simulink subsystem "i2c_slave_serializer"  (R2022b)
settings: Solver=VariableStepAuto  StartTime=0.0  StopTime=10.0  RelTol=1e-3
libraries: hdlsllib x20, simulink x18
Description:
  | //////////////////////////////////////////////////////////////////////
  | ////                                                              ////
  | //// serialInterface.v                                                 ////
  | ////                                                              ////
  | //// This file is part of the i2cSlave opencores effort.
  | //// <http://www.opencores.org/cores//>                           ////
  | ////                                                              ////
  | //// Module Description:                                          ////
  | //// Perform all serial to parallel, and parallel
  | //// to serial conversions. Perform device address matching
  | //// Handle arbitrary length I2C reads terminated by NAK
  | //// from host, and arbitrary length I2C writes terminated
  | //// by STOP from host
  | //// The second byte of a I2C write is always interpreted
  | //// as a register address, and becomes the base register address
  | //// for all read and write transactions.
  | //// I2C WRITE:    devAddr, regAddr, data[regAddr], data[regAddr+1], ..... data[regAddr+N]
  | //// I2C READ:    data[regAddr], data[regAddr+1], ..... data[regAddr+N]
  | //// Note that when regAddR reaches 255 it will automatically wrap round to 0
  | ////                                                              ////
  | //// To Do:                                                       ////
  | ////
  | ////                                                              ////
  | //// Author(s):                                                   ////
  | //// - Steve Fielding, sfielding@base2designs.com                 ////
  | ////                                                              ////
  | //////////////////////////////////////////////////////////////////////
  | ////                                                              ////
  | //// Copyright (C) 2008 Steve Fielding and OPENCORES.ORG          ////
  | ////                                                              ////
  | //// This source file may be used and distributed without         ////
  | //// restriction provided that this copyright statement is not    ////
  | //// removed from the file and that any derivative work contains  ////
  | //// the original copyright notice and the associated disclaimer. ////
  | ////                                                              ////
  | //// This source file is free software; you can redistribute it   ////
  | //// and/or modify it under the terms of the GNU Lesser General   ////
  | //// Public License as published by the Free Software Foundation; ////
  | //// either version 2.1 of the License, or (at your option) any   ////
  | //// later version.                                               ////
  | ////                                                              ////
  | //// This source is distributed in the hope that it will be       ////
  | //// useful, but WITHOUT ANY WARRANTY; without even the implied   ////
  | //// warranty of MERCHANTABILITY or FITNESS FOR A PARTICULAR      ////
  | //// PURPOSE. See the GNU Lesser General Public License for more  ////
  | //// details.                                                     ////
  | ////                                                              ////
  | //// You should have received a copy of the GNU Lesser General    ////
  | //// Public License along with this source; if not, download it   ////
  | //// from <http://www.opencores.org/lgpl.shtml>                   ////
  | ////                                                              ////
  | //////////////////////////////////////////////////////////////////////
settings Model: Creator=evsenin  LastModifiedBy=evsenin
settings ModelReferenceCC: EnableRefExpFcnMdlSchedulingChecks=on

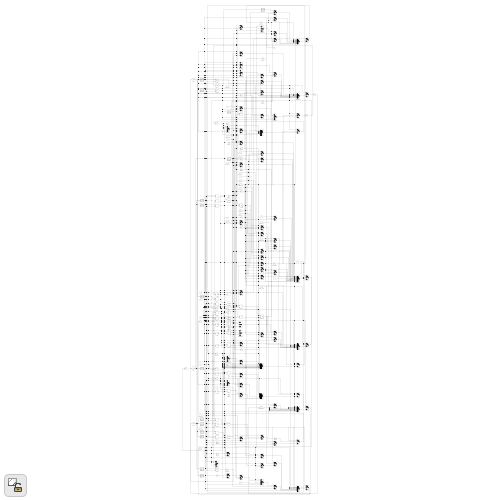
[thumbnail: Simulink's stored preview of the top-level diagram]
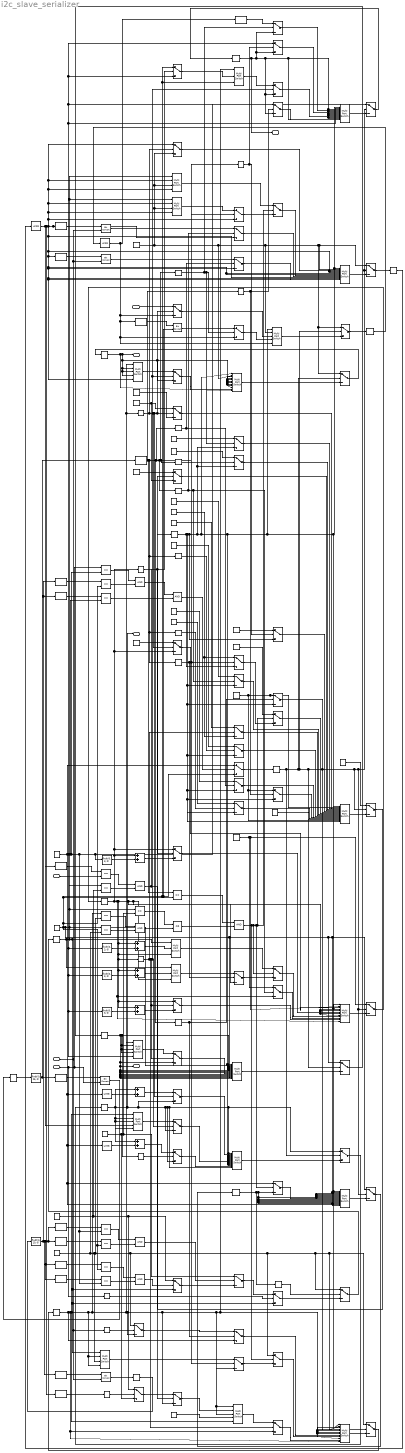
== system i2c_slave_serializer ==
  scl : Inport  OutDataTypeStr=fixdt(0, 1, 0)  SampleTime=-1
  sdaIn : Inport  Port=2  OutDataTypeStr=fixdt(0, 1, 0)  SampleTime=-1
  dataIn : Inport  Port=3  OutDataTypeStr=uint8  SampleTime=-1
  I2C_ADDRESS : Inport  Port=4  OutDataTypeStr=fixdt(0, 7, 0)  SampleTime=-1
  Add : Sum  AccumDataTypeStr=fixdt(0, 3, 0)  OutDataTypeStr=fixdt(0, 3, 0)  SampleTime=-1
  Add_1 : Sum  AccumDataTypeStr=fixdt(0, 3, 0)  OutDataTypeStr=fixdt(0, 3, 0)  SampleTime=-1
  Add_2 : Sum  AccumDataTypeStr=fixdt(0, 3, 0)  OutDataTypeStr=fixdt(0, 3, 0)  SampleTime=-1
  Add_3 : Sum  AccumDataTypeStr=fixdt(0, 3, 0)  OutDataTypeStr=fixdt(0, 3, 0)  SampleTime=-1
  Add_4 : Sum  AccumDataTypeStr=uint8  OutDataTypeStr=uint8  SampleTime=-1
  Add_5 : Sum  AccumDataTypeStr=uint8  OutDataTypeStr=uint8  SampleTime=-1
  Bit_Slice : hdlsllib/Logic and Bit Operations/Bit Slice  lidx=double(23)  ridx=double(0)
  Bit_Slice_1 : hdlsllib/Logic and Bit Operations/Bit Slice  lidx=double(8)  ridx=double(0)
  Bit_Slice_10 : hdlsllib/Logic and Bit Operations/Bit Slice  lidx=double(0)  ridx=double(0)
  Bit_Slice_11 : hdlsllib/Logic and Bit Operations/Bit Slice  lidx=double(6)  ridx=double(0)
  Bit_Slice_12 : hdlsllib/Logic and Bit Operations/Bit Slice  lidx=double(6)  ridx=double(0)
  Bit_Slice_13 : hdlsllib/Logic and Bit Operations/Bit Slice  lidx=double(6)  ridx=double(0)
  Bit_Slice_14 : hdlsllib/Logic and Bit Operations/Bit Slice  lidx=double(7)  ridx=double(7)
  Bit_Slice_2 : hdlsllib/Logic and Bit Operations/Bit Slice  lidx=double(24)  ridx=double(24)
  Bit_Slice_3 : hdlsllib/Logic and Bit Operations/Bit Slice  lidx=double(8)  ridx=double(8)
  Bit_Slice_4 : hdlsllib/Logic and Bit Operations/Bit Slice  lidx=double(9)  ridx=double(9)
  Bit_Slice_5 : hdlsllib/Logic and Bit Operations/Bit Slice  lidx=double(8)  ridx=double(8)
  Bit_Slice_6 : hdlsllib/Logic and Bit Operations/Bit Slice  lidx=double(9)  ridx=double(9)
  Bit_Slice_7 : hdlsllib/Logic and Bit Operations/Bit Slice  lidx=double(8)  ridx=double(8)
  Bit_Slice_8 : hdlsllib/Logic and Bit Operations/Bit Slice  lidx=double(9)  ridx=double(9)
  Bit_Slice_9 : hdlsllib/Logic and Bit Operations/Bit Slice  lidx=double(7)  ridx=double(1)
  CONST_u1b_0 : Constant  Value=0  OutDataTypeStr=fixdt(0, 1, 0)  SampleTime=-1
  CONST_u1b_1 : Constant  OutDataTypeStr=fixdt(0, 1, 0)  SampleTime=-1
  CONST_u2b_00 : Constant  Value=0  OutDataTypeStr=fixdt(0, 2, 0)  SampleTime=-1
  CONST_u2b_01 : Constant  OutDataTypeStr=fixdt(0, 2, 0)  SampleTime=-1
  CONST_u2b_10 : Constant  Value=2  OutDataTypeStr=fixdt(0, 2, 0)  SampleTime=-1
  CONST_u2b_11 : Constant  Value=3  OutDataTypeStr=fixdt(0, 2, 0)  SampleTime=-1
  CONST_u3b_000 : Constant  Value=0  OutDataTypeStr=fixdt(0, 3, 0)  SampleTime=-1
  CONST_u3b_001 : Constant  OutDataTypeStr=fixdt(0, 3, 0)  SampleTime=-1
  CONST_u4b_0000 : Constant  Value=0  OutDataTypeStr=fixdt(0, 4, 0)  SampleTime=-1
  CONST_u4b_0001 : Constant  OutDataTypeStr=fixdt(0, 4, 0)  SampleTime=-1
  CONST_u4b_0010 : Constant  Value=2  OutDataTypeStr=fixdt(0, 4, 0)  SampleTime=-1
  CONST_u4b_0011 : Constant  Value=3  OutDataTypeStr=fixdt(0, 4, 0)  SampleTime=-1
  CONST_u4b_0100 : Constant  Value=4  OutDataTypeStr=fixdt(0, 4, 0)  SampleTime=-1
  CONST_u4b_0101 : Constant  Value=5  OutDataTypeStr=fixdt(0, 4, 0)  SampleTime=-1
  CONST_u4b_0110 : Constant  Value=6  OutDataTypeStr=fixdt(0, 4, 0)  SampleTime=-1
  CONST_u4b_0111 : Constant  Value=7  OutDataTypeStr=fixdt(0, 4, 0)  SampleTime=-1
  CONST_u4b_1000 : Constant  Value=8  OutDataTypeStr=fixdt(0, 4, 0)  SampleTime=-1
  CONST_u4b_1001 : Constant  Value=9  OutDataTypeStr=fixdt(0, 4, 0)  SampleTime=-1
  CONST_u4b_1010 : Constant  Value=10  OutDataTypeStr=fixdt(0, 4, 0)  SampleTime=-1
  CONST_u4b_1011 : Constant  Value=11  OutDataTypeStr=fixdt(0, 4, 0)  SampleTime=-1
  CONST_u4b_1100 : Constant  Value=12  OutDataTypeStr=fixdt(0, 4, 0)  SampleTime=-1
  CONST_u4b_1101 : Constant  Value=13  OutDataTypeStr=fixdt(0, 4, 0)  SampleTime=-1
  CONST_u4b_1110 : Constant  Value=14  OutDataTypeStr=fixdt(0, 4, 0)  SampleTime=-1
  CONST_u4b_1111 : Constant  Value=15  OutDataTypeStr=fixdt(0, 4, 0)  SampleTime=-1
  CONST_u8b_00 : Constant  Value=0  OutDataTypeStr=uint8  SampleTime=-1
  Concat : hdlsllib/Logic and Bit Operations/Bit Concat  numInputs=2
  Concat_{1..4} (4 alike) : hdlsllib/Logic and Bit Operations/Bit Concat  numInputs=2
  CurrState_SISt_reg : Delay  DelayLength=double(1)  InitialCondition=0  SampleTime=-1
  Eq : RelationalOperator  Operator===  OutDataTypeStr=fixdt(0,1,0)  SampleTime=-1  InputSameDT=off
  Eq_{1..2,5..8,11..14,17..18} (12 alike) : RelationalOperator  Operator===  OutDataTypeStr=fixdt(0,1,0)  SampleTime=-1  InputSameDT=off
  Logical_AND : Logic  AllPortsSameDT=off  OutDataTypeStr=fixdt(0, 1, 0)  SampleTime=-1
  Logical_AND_{1..6} (6 alike) : Logic  AllPortsSameDT=off  OutDataTypeStr=fixdt(0, 1, 0)  SampleTime=-1
  Logical_OR : Logic  Operator=OR  AllPortsSameDT=off  OutDataTypeStr=fixdt(0, 1, 0)  SampleTime=-1
  MultiPortSwitch : MultiPortSwitch  DataPortOrder=Zero-based contiguous  Inputs=11  DiagnosticForDefault=None  zeroidx=on  OutDataTypeStr=fixdt(0, 2, 0)  SampleTime=-1  SaturateOnIntegerOverflow=off  InputSameDT=off
  MultiPortSwitch_1 : MultiPortSwitch  DataPortOrder=Zero-based contiguous  DiagnosticForDefault=None  zeroidx=on  OutDataTypeStr=fixdt(0, 2, 0)  SampleTime=-1  SaturateOnIntegerOverflow=off  InputSameDT=off
  MultiPortSwitch_10 : MultiPortSwitch  DataPortOrder=Zero-based contiguous  Inputs=4  DiagnosticForDefault=None  zeroidx=on  OutDataTypeStr=fixdt(0, 1, 0)  SampleTime=-1  SaturateOnIntegerOverflow=off  InputSameDT=off
  MultiPortSwitch_11 : MultiPortSwitch  DataPortOrder=Zero-based contiguous  Inputs=11  DiagnosticForDefault=None  zeroidx=on  OutDataTypeStr=uint8  SampleTime=-1  SaturateOnIntegerOverflow=off  InputSameDT=off
  MultiPortSwitch_12 : MultiPortSwitch  DataPortOrder=Zero-based contiguous  Inputs=4  DiagnosticForDefault=None  zeroidx=on  OutDataTypeStr=uint8  SampleTime=-1  SaturateOnIntegerOverflow=off  InputSameDT=off
  MultiPortSwitch_13 : MultiPortSwitch  DataPortOrder=Zero-based contiguous  Inputs=11  DiagnosticForDefault=None  zeroidx=on  OutDataTypeStr=fixdt(0, 3, 0)  SampleTime=-1  SaturateOnIntegerOverflow=off  InputSameDT=off
  MultiPortSwitch_14 : MultiPortSwitch  DataPortOrder=Zero-based contiguous  Inputs=2  DiagnosticForDefault=None  zeroidx=on  OutDataTypeStr=fixdt(0, 3, 0)  SampleTime=-1  SaturateOnIntegerOverflow=off  InputSameDT=off
  MultiPortSwitch_15 : MultiPortSwitch  DataPortOrder=Zero-based contiguous  Inputs=2  DiagnosticForDefault=None  zeroidx=on  OutDataTypeStr=fixdt(0, 3, 0)  SampleTime=-1  SaturateOnIntegerOverflow=off  InputSameDT=off
  MultiPortSwitch_16 : MultiPortSwitch  DataPortOrder=Zero-based contiguous  Inputs=16  DiagnosticForDefault=None  zeroidx=on  OutDataTypeStr=fixdt(0, 1, 0)  SampleTime=-1  SaturateOnIntegerOverflow=off  InputSameDT=off
  MultiPortSwitch_17 : MultiPortSwitch  DataPortOrder=Zero-based contiguous  Inputs=16  DataPortForDefault=Additional data port  DiagnosticForDefault=None  zeroidx=on  OutDataTypeStr=fixdt(0, 4, 0)  SampleTime=-1  SaturateOnIntegerOverflow=off  InputSameDT=off
  MultiPortSwitch_18 : MultiPortSwitch  DataPortOrder=Zero-based contiguous  Inputs=16  DiagnosticForDefault=None  zeroidx=on  OutDataTypeStr=uint8  SampleTime=-1  SaturateOnIntegerOverflow=off  InputSameDT=off
  MultiPortSwitch_19 : MultiPortSwitch  DataPortOrder=Zero-based contiguous  Inputs=4  DiagnosticForDefault=None  zeroidx=on  OutDataTypeStr=uint8  SampleTime=-1  SaturateOnIntegerOverflow=off  InputSameDT=off
  MultiPortSwitch_2 : MultiPortSwitch  DataPortOrder=Zero-based contiguous  Inputs=4  DiagnosticForDefault=None  zeroidx=on  OutDataTypeStr=fixdt(0, 2, 0)  SampleTime=-1  SaturateOnIntegerOverflow=off  InputSameDT=off
  MultiPortSwitch_3 : MultiPortSwitch  DataPortOrder=Zero-based contiguous  Inputs=4  DiagnosticForDefault=None  zeroidx=on  OutDataTypeStr=uint8  SampleTime=-1  SaturateOnIntegerOverflow=off  InputSameDT=off
  MultiPortSwitch_4 : MultiPortSwitch  DataPortOrder=Zero-based contiguous  Inputs=13  DiagnosticForDefault=None  zeroidx=on  OutDataTypeStr=uint8  SampleTime=-1  SaturateOnIntegerOverflow=off  InputSameDT=off
  MultiPortSwitch_5 : MultiPortSwitch  DataPortOrder=Zero-based contiguous  DiagnosticForDefault=None  zeroidx=on  OutDataTypeStr=uint8  SampleTime=-1  SaturateOnIntegerOverflow=off  InputSameDT=off
  MultiPortSwitch_6 : MultiPortSwitch  DataPortOrder=Zero-based contiguous  DiagnosticForDefault=None  zeroidx=on  OutDataTypeStr=uint8  SampleTime=-1  SaturateOnIntegerOverflow=off  InputSameDT=off
  MultiPortSwitch_7 : MultiPortSwitch  DataPortOrder=Zero-based contiguous  Inputs=14  DiagnosticForDefault=None  zeroidx=on  OutDataTypeStr=fixdt(0, 1, 0)  SampleTime=-1  SaturateOnIntegerOverflow=off  InputSameDT=off
  MultiPortSwitch_8 : MultiPortSwitch  DataPortOrder=Zero-based contiguous  Inputs=2  DiagnosticForDefault=None  zeroidx=on  OutDataTypeStr=fixdt(0, 1, 0)  SampleTime=-1  SaturateOnIntegerOverflow=off  InputSameDT=off
  MultiPortSwitch_9 : MultiPortSwitch  DataPortOrder=Zero-based contiguous  Inputs=16  DiagnosticForDefault=None  zeroidx=on  OutDataTypeStr=fixdt(0, 1, 0)  SampleTime=-1  SaturateOnIntegerOverflow=off  InputSameDT=off
  RelEQ191 : simulink/Logic and Bit Operations/Compare To Constant  relop===  const="fi(0,0,1,0,\"hex\",\"1\")"  OutDataTypeStr=boolean
  RelEQ197 : simulink/Logic and Bit Operations/Compare To Constant  relop===  const="fi(0,0,1,0,\"hex\",\"1\")"  OutDataTypeStr=boolean
  RelEQ_127 : simulink/Logic and Bit Operations/Compare To Constant  relop===  const="fi(0,0,2,0,\"hex\",\"1\")"  OutDataTypeStr=boolean
  RelEQ_{149,182,232,357,372} (5 alike) : simulink/Logic and Bit Operations/Compare To Constant  relop===  const="fi(0,0,1,0,\"hex\",\"0\")"  OutDataTypeStr=boolean
  RelEQ_{165,191,193,273,297,362,382,387} (8 alike) : simulink/Logic and Bit Operations/Compare To Constant  relop===  const="fi(0,0,1,0,\"hex\",\"1\")"  OutDataTypeStr=boolean
  RelEQ_171 : simulink/Logic and Bit Operations/Compare To Constant  relop===  const="fi(0,0,3,0,\"hex\",\"0\")"  OutDataTypeStr=boolean
  RelEQ_287 : simulink/Logic and Bit Operations/Compare To Constant  relop===  const="fi(0,0,3,0,\"hex\",\"7\")"  OutDataTypeStr=boolean
  Switch : Switch  Criteria=u2 ~= 0  Threshold=double(0)  OutDataTypeStr=fixdt(0, 1, 0)  SampleTime=-1  SaturateOnIntegerOverflow=off  InputSameDT=off
  Switch_{1..11,55} (12 alike) : Switch  Criteria=u2 ~= 0  Threshold=double(0)  OutDataTypeStr=fixdt(0, 2, 0)  SampleTime=-1  SaturateOnIntegerOverflow=off  InputSameDT=off
  Switch_{12..18,25,47..49,53,56..57,59} (15 alike) : Switch  Criteria=u2 ~= 0  Threshold=double(0)  OutDataTypeStr=uint8  SampleTime=-1  SaturateOnIntegerOverflow=off  InputSameDT=off
  Switch_{19..24,32,51..52,54} (10 alike) : Switch  Criteria=u2 ~= 0  Threshold=double(0)  OutDataTypeStr=fixdt(0, 1, 0)  SampleTime=-1  SaturateOnIntegerOverflow=off  InputSameDT=off
  Switch_{26..31,58} (7 alike) : Switch  Criteria=u2 ~= 0  Threshold=double(0)  OutDataTypeStr=fixdt(0, 3, 0)  SampleTime=-1  SaturateOnIntegerOverflow=off  InputSameDT=off
  Switch_{33..46,50} (15 alike) : Switch  Criteria=u2 ~= 0  Threshold=double(0)  OutDataTypeStr=fixdt(0, 4, 0)  SampleTime=-1  SaturateOnIntegerOverflow=off  InputSameDT=off
  bitCnt_reg : Delay  DelayLength=double(1)  InitialCondition=0  SampleTime=-1
  clearStartStopDet_reg : Delay  DelayLength=double(1)  InitialCondition=0  SampleTime=-1
  dataOut_1_reg : Delay  DelayLength=double(1)  InitialCondition=0  SampleTime=-1
  dtc{,1..3} (4 alike) : DataTypeConversion  OutDataTypeStr=fixdt(0, 3, 0)  SampleTime=-1  SaturateOnIntegerOverflow=off  RndMeth=Floor
  dtc{4..7} (4 alike) : DataTypeConversion  OutDataTypeStr=uint8  SampleTime=-1  SaturateOnIntegerOverflow=off  RndMeth=Floor
  dtc8 : DataTypeConversion  OutDataTypeStr=fixdt(0, 25, 0)  SampleTime=-1  SaturateOnIntegerOverflow=off  RndMeth=Floor
  dtc9 : DataTypeConversion  OutDataTypeStr=fixdt(0, 10, 0)  SampleTime=-1  SaturateOnIntegerOverflow=off  RndMeth=Floor
  regAddr_1_reg : Delay  DelayLength=double(1)  InitialCondition=0  SampleTime=-1
  rxData_reg : Delay  DelayLength=double(1)  InitialCondition=0  SampleTime=-1
  sclDelayed_reg : Delay  DelayLength=double(1)  InitialCondition=0  SampleTime=-1
  sdaDelayed_reg : Delay  DelayLength=double(1)  InitialCondition=0  SampleTime=-1
  sdaOut_1_reg : Delay  DelayLength=double(1)  InitialCondition=1  SampleTime=-1
  startEdgeDet_reg : Delay  DelayLength=double(1)  InitialCondition=0  SampleTime=-1
  startStopDetState_reg : Delay  DelayLength=double(1)  InitialCondition=0  SampleTime=-1
  streamSt_reg : Delay  DelayLength=double(1)  InitialCondition=0  SampleTime=-1
  txData_reg : Delay  DelayLength=double(1)  InitialCondition=0  SampleTime=-1
  writeEn_1_reg : Delay  DelayLength=double(1)  InitialCondition=0  SampleTime=-1
  sdaOut : Outport  OutDataTypeStr=fixdt(0, 1, 0)  SampleTime=-1
  dataOut : Outport  Port=2  OutDataTypeStr=uint8  SampleTime=-1
  regAddr : Outport  Port=3  OutDataTypeStr=uint8  SampleTime=-1
  writeEn : Outport  Port=4  OutDataTypeStr=fixdt(0, 1, 0)  SampleTime=-1
  wires:
  Switch_32/1 -> MultiPortSwitch_16/9
  dtc3/1 -> Add_3/2
  MultiPortSwitch_11/1 -> Switch_53/3
  Switch_58/1 -> bitCnt_reg/1
  MultiPortSwitch/1 -> Switch_55/3
  Switch/1 -> startEdgeDet_reg/1
  Switch_50/1 -> CurrState_SISt_reg/1
  CONST_u3b_001/1 -> Switch_26/1
  Switch_29/1 -> Switch_28/3
  Logical_AND_3/1 -> Switch_4/2
  CONST_u4b_0101/1 -> Switch_36/1
  RelEQ197/1 -> Switch_2/2
  Eq_8/1 -> Logical_AND_3/2
  Eq_13/1 -> Logical_AND_5/1
  Switch_8/1 -> Switch_7/3
  MultiPortSwitch_19/1 -> Switch_48/1
  Eq_14/1 -> Logical_AND_5/2
  Switch_4/1 -> Switch_3/3
  Switch_24/1 -> MultiPortSwitch_9/11
  Switch_42/1 -> MultiPortSwitch_17/11
  Concat_3/1 -> Switch_17/1
  MultiPortSwitch_1/1 -> Switch_8/1
  RelEQ_297/1 -> Switch_11/2
  Switch_28/1 -> MultiPortSwitch_13/9
  Switch_15/1 -> MultiPortSwitch_4/9
  RelEQ_193/1 -> Switch_6/2
  Switch_12/1 -> MultiPortSwitch_3/3
  Switch_34/1 -> MultiPortSwitch_17/4
  Bit_Slice_10/1 -> RelEQ_297/1
  Switch_41/1 -> MultiPortSwitch_17/10
  Switch_47/1 -> MultiPortSwitch_18/3
  Switch_20/1 -> MultiPortSwitch_7/7
  Concat_4/1 -> Switch_18/1
  Switch_37/1 -> MultiPortSwitch_17/7
  RelEQ_382/1 -> Switch_46/2
  Bit_Slice_14/1 -> Switch_19/1
  Switch_19/1 -> MultiPortSwitch_7/4
  bitCnt_reg/1 -> Add/1, Switch_27/1, Switch_26/3, RelEQ_171/1, Switch_29/3, MultiPortSwitch_15/3, MultiPortSwitch_13/4, MultiPortSwitch_13/5, MultiPortSwitch_13/7, MultiPortSwitch_13/8, Add_1/1, MultiPortSwitch_14/3, RelEQ_287/1, Add_2/1, Switch_31/1, Add_3/1, MultiPortSwitch_13/12, Switch_30/3
  CONST_u2b_10/1 -> Switch_11/3, Switch_3/1, Eq_12/2
  Switch_30/1 -> MultiPortSwitch_13/10
  CONST_u4b_1010/1 -> Switch_44/1
  Eq/1 -> Logical_AND_1/1
  Eq_17/1 -> Logical_AND_6/1
  RelEQ_387/1 -> Switch_49/2
  RelEQ_171/1 -> Switch_27/2, Switch_36/2
  Eq_2/1 -> Logical_AND/2
  Logical_OR/1 -> Logical_AND_4/2
  Logical_AND_6/1 -> Switch_10/2, Switch_22/2
  dtc2/1 -> Add_2/2
  dtc4/1 -> Add_4/2
  Eq_6/1 -> Logical_AND_2/2
  Switch_59/1 -> regAddr_1_reg/1
  RelEQ_273/1 -> Switch_17/2, Switch_30/2, Switch_41/2
  Eq_12/1 -> Logical_OR/1
  Switch_2/1 -> Switch_1/3
  MultiPortSwitch_2/1 -> Switch_9/1
  Switch_55/1 -> streamSt_reg/1
  Switch_31/1 -> MultiPortSwitch_13/11
  Switch_16/1 -> Switch_15/3
  Switch_18/1 -> MultiPortSwitch_4/13
  Switch_53/1 -> dataOut_1_reg/1
  Switch_11/1 -> Switch_10/1
  I2C_ADDRESS/1 -> Eq_17/2
  Logical_AND_2/1 -> Switch_3/2
  clearStartStopDet_reg/1 -> RelEQ191/1, Switch_32/3, MultiPortSwitch_16/8, MultiPortSwitch_16/7, MultiPortSwitch_16/6, MultiPortSwitch_16/5, MultiPortSwitch_16/3, MultiPortSwitch_16/4, MultiPortSwitch_16/10, MultiPortSwitch_16/11, MultiPortSwitch_16/12, MultiPortSwitch_16/13, MultiPortSwitch_16/14
  Bit_Slice_8/1 -> Eq_8/1
  Switch_54/1 -> clearStartStopDet_reg/1
  CONST_u4b_0000/1 -> Switch_50/1
  CONST_u4b_1110/1 -> Switch_42/1
  scl/1 -> RelEQ197/1, Concat/2, Eq/1
  Switch_56/1 -> txData_reg/1
  Switch_23/1 -> MultiPortSwitch_7/14
  Switch_21/1 -> MultiPortSwitch_7/11
  CurrState_SISt_reg/1 -> Switch_40/3, MultiPortSwitch_17/18, Switch_37/3, Switch_34/3, Switch_35/3, MultiPortSwitch_11/1, MultiPortSwitch_3/1, MultiPortSwitch_17/1, MultiPortSwitch_4/1, MultiPortSwitch_7/1, MultiPortSwitch_13/1, MultiPortSwitch/1, MultiPortSwitch_16/1, MultiPortSwitch_9/1, MultiPortSwitch_18/1, Switch_41/3, Switch_38/3, Switch_43/3, Switch_44/3, Switch_45/3, Switch_46/3
  Bit_Slice_7/1 -> Eq_7/1
  sdaIn/1 -> Concat_3/2, Concat_4/2, Concat_1/2, RelEQ_193/1
  CONST_u1b_0/1 -> Eq_1/2, Eq_11/2, MultiPortSwitch_8/3, Switch_22/1, Switch/3, Concat_2/2, MultiPortSwitch_9/2, MultiPortSwitch_9/16, Switch_52/1, Switch_54/1, MultiPortSwitch_16/2, MultiPortSwitch_16/15, MultiPortSwitch_16/17, Eq_6/2, Eq_7/2
  CONST_u1b_1/1 -> Switch/1, MultiPortSwitch_7/2, Switch_23/1, Switch_20/1, Switch_22/3, Eq_2/2, Eq/2, dtc/1, Switch_51/1, Eq_5/2, Eq_8/2, dtc1/1, dtc2/1, MultiPortSwitch_10/5, dtc3/1, dtc4/1, dtc5/1, MultiPortSwitch_16/16, Switch_32/1
  Concat/1 -> sclDelayed_reg/1
  Bit_Slice_12/1 -> Concat_3/1
  CONST_u4b_0001/1 -> MultiPortSwitch_17/2, Switch_38/1, MultiPortSwitch_17/17, Switch_45/1
  RelEQ_357/1 -> Switch_43/2
  Logical_AND/1 -> Switch/2
  CONST_u4b_0010/1 -> Switch_33/1, Switch_36/3
  RelEQ_362/1 -> Switch_18/2, Switch_44/2
  Switch_52/1 -> writeEn_1_reg/1
  RelEQ_127/1 -> Switch_14/2, Switch_26/2, Switch_47/2, Switch_12/2, Switch_33/2
  MultiPortSwitch_16/1 -> Switch_54/3
  MultiPortSwitch_18/1 -> Switch_59/3
  Add_4/1 -> Switch_47/1
  CONST_u2b_00/1 -> Eq_14/2, MultiPortSwitch_1/3, Eq_13/2, Switch_6/1, Switch_7/1, Switch_1/1, MultiPortSwitch/2, Switch_55/1
  MultiPortSwitch_6/1 -> Switch_16/1
  Bit_Slice_1/1 -> Concat_1/1
  MultiPortSwitch_12/1 -> Switch_25/1
  Bit_Slice_6/1 -> Eq_6/1
  Switch_35/1 -> MultiPortSwitch_17/5
  sdaOut_1_reg/1 -> sdaOut/1, Switch_19/3, Switch_20/3, MultiPortSwitch_7/15, MultiPortSwitch_7/3, MultiPortSwitch_7/5, MultiPortSwitch_7/6, MultiPortSwitch_7/8, MultiPortSwitch_7/9, MultiPortSwitch_7/10, MultiPortSwitch_7/12, MultiPortSwitch_7/13, Switch_21/3, Switch_23/3
  Add_5/1 -> Switch_49/1
  Switch_39/1 -> MultiPortSwitch_17/9
  CONST_u4b_0100/1 -> Switch_35/1
  rxData_reg/1 -> dtc6/1
  RelEQ_165/1 -> Switch_35/2
  CONST_u4b_0111/1 -> Switch_41/1
  Switch_26/1 -> MultiPortSwitch_13/3
  Switch_38/1 -> MultiPortSwitch_17/8
  CONST_u4b_1001/1 -> Switch_43/1
  CONST_u4b_1111/1 -> Switch_39/1
  Switch_49/1 -> MultiPortSwitch_18/16
  Switch_46/1 -> MultiPortSwitch_17/15
  Logical_AND_5/1 -> Logical_OR/2
  Eq_7/1 -> Logical_AND_3/1
  Switch_44/1 -> MultiPortSwitch_17/13
  Switch_25/1 -> MultiPortSwitch_11/11
  dtc1/1 -> Add_1/2
  Add_2/1 -> MultiPortSwitch_15/2
  Switch_27/1 -> MultiPortSwitch_13/6
  Bit_Slice_3/1 -> Eq_1/1
  CONST_u4b_1100/1 -> Switch_46/1
  Eq_18/1 -> Logical_AND_6/2
  Switch_43/1 -> MultiPortSwitch_17/12
  Switch_3/1 -> Switch_2/1
  sdaDelayed_reg/1 -> dtc9/1
  CONST_u4b_0110/1 -> Switch_37/1
  txData_reg/1 -> dtc7/1
  sclDelayed_reg/1 -> dtc8/1
  CONST_u4b_1101/1 -> MultiPortSwitch_17/16
  regAddr_1_reg/1 -> Add_4/1, Add_5/1, regAddr/1, Switch_47/3, Switch_48/3, Switch_49/3, MultiPortSwitch_18/17, Switch_59/1, MultiPortSwitch_18/2, MultiPortSwitch_18/4, MultiPortSwitch_18/5, MultiPortSwitch_18/6, MultiPortSwitch_18/7, MultiPortSwitch_18/8, MultiPortSwitch_18/9, MultiPortSwitch_18/10, MultiPortSwitch_18/12, MultiPortSwitch_18/13, MultiPortSwitch_18/14, MultiPortSwitch_18/15, MultiPortSwitch_19/2, MultiPortSwitch_19/3, MultiPortSwitch_19/5
  Switch_48/1 -> MultiPortSwitch_18/11
  Switch_9/1 -> MultiPortSwitch/11
  CONST_u4b_0011/1 -> Switch_34/1
  Bit_Slice_2/1 -> RelEQ_372/1, Eq_11/1, RelEQ_191/1, RelEQ_362/1, RelEQ_273/1, RelEQ_149/1, RelEQ_182/1, RelEQ_165/1, RelEQ_357/1, RelEQ_232/1, RelEQ_382/1
  Eq_5/1 -> Logical_AND_2/1
  CONST_u3b_000/1 -> Switch_30/1, MultiPortSwitch_13/2, Switch_58/1
  CONST_u4b_1000/1 -> Switch_33/3
  Eq_11/1 -> Logical_AND_4/1
  dataOut_1_reg/1 -> MultiPortSwitch_11/12, dataOut/1, Switch_25/3, MultiPortSwitch_11/3, MultiPortSwitch_11/4, MultiPortSwitch_11/5, MultiPortSwitch_11/6, MultiPortSwitch_11/7, MultiPortSwitch_11/8, MultiPortSwitch_11/9, MultiPortSwitch_11/10, MultiPortSwitch_12/2, MultiPortSwitch_12/3, MultiPortSwitch_12/4
  Switch_10/1 -> MultiPortSwitch_2/2
  Bit_Slice_4/1 -> Eq_2/1
  Switch_1/1 -> startStopDetState_reg/1
  Switch_17/1 -> MultiPortSwitch_4/10
  MultiPortSwitch_8/1 -> Switch_21/1
  writeEn_1_reg/1 -> RelEQ_387/1, MultiPortSwitch_9/3, MultiPortSwitch_9/4, MultiPortSwitch_9/5, MultiPortSwitch_9/6, MultiPortSwitch_9/7, MultiPortSwitch_10/2, MultiPortSwitch_10/3, MultiPortSwitch_10/4, Switch_24/3, writeEn/1, MultiPortSwitch_9/8, MultiPortSwitch_9/9, MultiPortSwitch_9/10, MultiPortSwitch_9/12, MultiPortSwitch_9/13, MultiPortSwitch_9/14, MultiPortSwitch_9/15, MultiPortSwitch_9/17
  Bit_Slice_5/1 -> Eq_5/1
  RelEQ_232/1 -> Switch_29/2, Switch_8/2, Switch_16/2, Switch_40/2
  MultiPortSwitch_13/1 -> Switch_58/3
  RelEQ_149/1 -> Switch_19/2, Switch_13/2, Switch_34/2
  dtc/1 -> Add/2
  MultiPortSwitch_10/1 -> Switch_24/1
  Logical_AND_1/1 -> Logical_AND/1
  dtc8/1 -> Bit_Slice/1, Bit_Slice_2/1
  dtc7/1 -> Bit_Slice_14/1, Switch_12/3, Bit_Slice_11/1, MultiPortSwitch_3/5, Switch_13/3
  Switch_7/1 -> MultiPortSwitch/9
  Bit_Slice/1 -> Concat/1
  Bit_Slice_9/1 -> Eq_17/1
  streamSt_reg/1 -> Switch_5/3, MultiPortSwitch_2/5, MultiPortSwitch_19/1, Eq_13/1, MultiPortSwitch_10/1, RelEQ_127/1, MultiPortSwitch_12/1, Switch_6/3, Switch_10/3, Switch_8/3, MultiPortSwitch_8/1, MultiPortSwitch/3, MultiPortSwitch/4, MultiPortSwitch/5, MultiPortSwitch/6, MultiPortSwitch/7, MultiPortSwitch/10, MultiPortSwitch_2/1, MultiPortSwitch_2/3, MultiPortSwitch_1/2, MultiPortSwitch_1/4, MultiPortSwitch/12, Switch_9/3
  CONST_u8b_00/1 -> MultiPortSwitch_6/3, Switch_14/3, MultiPortSwitch_5/3, MultiPortSwitch_11/2, MultiPortSwitch_3/2, MultiPortSwitch_4/2, Switch_57/1, Switch_53/1, Switch_56/1
  Switch_33/1 -> MultiPortSwitch_17/3
  dataIn/1 -> Switch_12/1
  MultiPortSwitch_3/1 -> Switch_56/3
  Switch_5/1 -> MultiPortSwitch/8
  Concat_2/1 -> Switch_13/1
  Switch_14/1 -> MultiPortSwitch_4/3
  Add_1/1 -> MultiPortSwitch_14/2
  MultiPortSwitch_9/1 -> Switch_52/3
  MultiPortSwitch_14/1 -> Switch_28/1
  Concat_1/1 -> sdaDelayed_reg/1
  MultiPortSwitch_17/1 -> Switch_50/3
  RelEQ_191/1 -> Switch_5/2, Switch_38/2
  Bit_Slice_11/1 -> Concat_2/1
  Switch_13/1 -> MultiPortSwitch_3/4
  Switch_57/1 -> rxData_reg/1
  CONST_u2b_11/1 -> MultiPortSwitch_2/4
  Add/1 -> Switch_27/3
  RelEQ_287/1 -> Switch_42/2, Switch_9/2, Switch_48/2, Switch_21/2, Switch_25/2, Switch_24/2, Switch_31/2
  MultiPortSwitch_4/1 -> Switch_57/3
  dtc5/1 -> Add_5/2
  Switch_22/1 -> MultiPortSwitch_8/2
  Switch_36/1 -> MultiPortSwitch_17/6
  MultiPortSwitch_7/1 -> Switch_51/3
  Switch_45/1 -> MultiPortSwitch_17/14
  RelEQ_372/1 -> Switch_23/2, Switch_45/2
  CONST_u4b_1011/1 -> Switch_40/1, Switch_42/3
  Logical_AND_4/1 -> Switch_7/2, Switch_28/2, Switch_32/2, Switch_15/2, Switch_39/2
  startStopDetState_reg/1 -> MultiPortSwitch_15/1, Eq_14/1, Eq_12/1, Eq_18/1, MultiPortSwitch_5/1, MultiPortSwitch_6/1, MultiPortSwitch_14/1, Switch_4/3, Switch_2/3, MultiPortSwitch_1/1
  RelEQ191/1 -> Switch_1/2
  Switch_40/1 -> Switch_39/3
  Add_3/1 -> Switch_31/3
  dtc6/1 -> MultiPortSwitch_19/4, Bit_Slice_9/1, Bit_Slice_10/1, Switch_16/3, MultiPortSwitch_6/4, MultiPortSwitch_6/2, MultiPortSwitch_5/4, Switch_14/1, MultiPortSwitch_5/2, Switch_17/3, Bit_Slice_12/1, MultiPortSwitch_4/11, MultiPortSwitch_4/4, MultiPortSwitch_4/5, MultiPortSwitch_4/6, Bit_Slice_13/1, MultiPortSwitch_4/7, MultiPortSwitch_4/8, Switch_18/3, MultiPortSwitch_4/12, MultiPortSwitch_4/14, MultiPortSwitch_12/5
  MultiPortSwitch_15/1 -> Switch_29/1
  dtc9/1 -> Bit_Slice_3/1, Bit_Slice_4/1, Bit_Slice_1/1, Bit_Slice_5/1, Bit_Slice_6/1, Bit_Slice_7/1, Bit_Slice_8/1
  Switch_6/1 -> Switch_5/1
  RelEQ_182/1 -> Switch_20/2, Switch_37/2
  Eq_1/1 -> Logical_AND_1/2
  Switch_51/1 -> sdaOut_1_reg/1
  startEdgeDet_reg/1 -> Switch_59/2, Switch_53/2, Switch_56/2, Switch_52/2, Switch_55/2, Switch_50/2, Switch_51/2, Switch_57/2, Switch_54/2, Switch_58/2
  CONST_u2b_01/1 -> Eq_18/2, Switch_4/1, Switch_11/1
  MultiPortSwitch_5/1 -> Switch_15/1
  Bit_Slice_13/1 -> Concat_4/1
